simulink model "incubator_larma"  (R2023a)
settings: Solver=VariableStepAuto  StartTime=0.0  StopTime=10000  RelTol=1e-3
undefined symbols (not defined in the file or in its folder): Acv, Anet, Ar, As, Awi, bf, cp_b, cp_co, cpa, cpa_skin, cpm, cpw, eps_s, epsilon_w, Evap, hf_g, hfg, hien, hscv, IV, K_c, Kmat, kplex, m, ma, mco, ms, mw, Qmet, rho_a, rho_bl, rho_c, rho_w, Sa, sigma, th_w, thm, Wa, Wex
libraries: neural x1
settings Model: Creator=ACER  LastModifiedBy=ACER

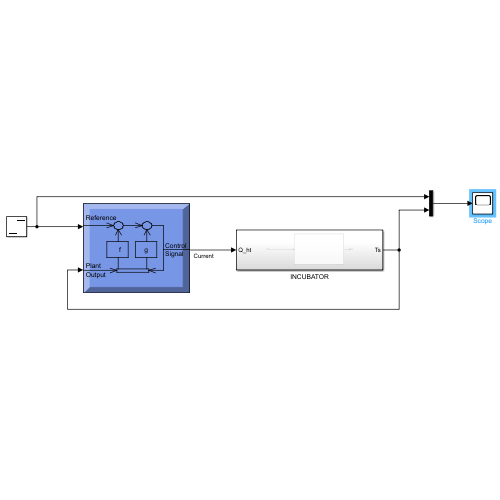
[thumbnail: Simulink's stored preview of the top-level diagram]
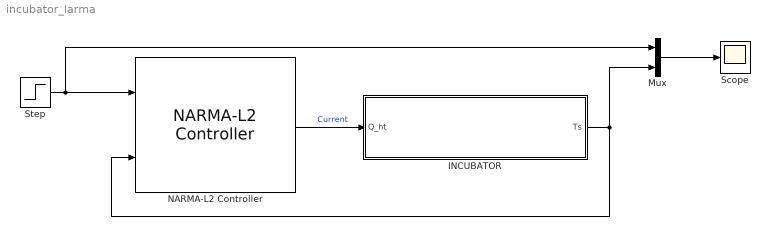
== system incubator_larma ==
  INCUBATOR : Subsystem
  Mux : Mux  Inputs=2
  NARMA-L2 Controller : neural/Control Systems/NARMA-L2 Controller  Normalize=0  IW1_1=[0.55311527878139377101 0.5598203760437183707;0.46124325685294664812 -0.0015039561193254337348;0.35378378182192637968 -0.017778723358536991511;-0.56208585013665313124 0.019429595098862040975;-0.74496852231229937491 -0.19223678100702804028;-0.18032373979217605764 -1.0804233481508331201e-05;-0.0282441180623933287 -1.9488745271411685823e-05;0.56561476199323101888 -0.048980800453075734602;-0.41624725454422795146 -2.9535601674756283214e-05;0.87246018830272520361 0.16107016027459286622;0.24117893087617620074 -0.0058257948908682806455;-0.69737494610867822864 -0.10448733539812102289;0.097948441462564567184 -0.019741652792315281251;0.57418035274274692448 -7.2088683216202652541e-05;0.5152796520885649656 -0.040344453154290062236;0.30918570905807551963 -0.021130285682796120378;-0.1040299484748695158 2.2106464471173243217e-06;-0.37176051328431147791 0.10309704107792808103;0.093748564233812642366 0.047052234342038257164;-0.54216462791611841343 -0.054531523988263504166;-0.42968180781873865914 0.055813498068482229886;0.55356647159035377026 0.04282325530096745686;0.36403213956220809022 -0.012973022507361995151;0.41088826816202883574 -0.10089012273490473304;0.46853931598860942831 -0.02420455926389125309;-0.41203096230894203922 -0.10280214872710646823;0.087678220875249249233 0.08967818975138343307;0.54183175861681087682 -0.00022750990821356916307;0.35782543615690320937 -0.041306439686633167341;0.63894568298766196701 0.14555547319291906039]  IW3_2=[-0.42869384870059590309 -0.20467390647117111868;0.54536161261206483886 0.0397307131399293606;-0.20380803372964173548 -0.093567928016329390828;-0.54440336065554817413 0.0017412995823690414175;0.41258415083026206416 -0.010924801743475522076;0.30671682947788436735 -0.0013301936152310287961;-0.30320085381841443972 0.06196663873638227904;-0.45125076837662364548 -0.0013054891628779591219;0.58589863417663268219 -0.009357661584803091126;0.22471210064158819719 0.036380518448993745539;-0.44856933606073828846 0.10557310034665394471;-0.52713778378582787365 -0.53957098764537259061;0.58612163553517704351 0.00012267588482581850409;0.20481716654358936291 0.099850170401508259177;-0.53543939332965750921 0.013380088910996708676;-0.55430247583245539911 0.00015211749869671132088;-0.060674901375614320731 0.0086928668514609716556;0.64518139636977545059 0.0055338968489383293103;-0.041112178189121904859 0.0015771853488393294297;0.069279982598140429917 0.080813967189555135917;0.0028529471897044108089 0.013322308884735010667;-0.41655325465272263763 -0.00403611729657711929;0.75859708272283676855 0.089147588049559495227;0.30545267983956803093 0.20601727557974147675;-0.55870608858082249082 0.010588837453492193699;0.074302051251215472938 0.0038643249470113908914;-0.00010236459103301481788 0.032472774763839959422;-0.23911146616137041176 0.019543603347508604895;0.084384658656527999909 -0.048307095295211939512;0.56830406068870620295 0.046981911977682609682]  IW5_3=0.093113430827311188809  LW2_1=[-1.7385414418328675179 1.185031400225210918 0.83172478025034168869 -1.4923108136193563578 0.86513570813376494684 0.55423887448822461987 -0.5403848605489650625 0.53040353884286517427 0.12742495894744695906 -2.0107365617688883752 1.7239949695213867553 1.456069982897223003 2.0136612826838233836 -1.927587542673245169 1.9384591441949254875 1.1335326599628925415 1.1219315777715177518 -1.487145524998456203 -1.9666798151412503426 1.8229411277316418527 -1.8311420627738832501 -1.3707653411339519867 1.3653022355198809468 2.1154712110253384161 1.1364878446942920931 2.1020303712400054685 -1.6675216724967341086 -0.027274724183782884934 1.3949442262661992942 -1.9913939889305762865]  LW4_3=[0.3597032512256021497 -0.63118082136266029369 0.37486171525082290223 -0.013348386024869672573 0.32965125262583028221 -0.79990641798758133074 -0.67897203390229565745 -0.18071553831118514211 0.14106801226241016955 -0.59570988892262688452 0.037331896445282973518 0.39855004856611631059 0.092510865835327929507 -0.23765480170884850653 -0.055617033718718608681 0.36860629457851767921 0.24445192286607583809 -0.37506410562211284221 0.65925844056717919361 -0.45477875753864865915 -0.30552264029698922299 -1.1194017489131884435 -0.11139933444262158091 -0.057504459052148286513 -0.25054450314805248867 -1.2495401767009046701 -0.37443973064932029038 1.4029097881644230217 0.57980235994644591102 -0.07556488017899547216]  LW5_4=-0.0053469523428589880304  LW6_5=0.97064188618752011983  LW6_2=-7.744036449301247238  B1=[-50.772852052828987723;-157.51505260377004447;-124.72206827114483474;183.33515481133116509;40.772018349078749111;57.712710053475049676;21.189182089565107958;-184.18249959630355761;135.3940445785350164;-179.3078176323155617;-85.609369809779011007;154.86499019897746621;-40.425578248012868698;-171.27574200038807817;-168.27088502237748457;-104.25105583651611596;31.911665330855385037;117.260366952972376;-18.822237201337674861;142.90914902327949676;147.83695329597799173;-160.21319473749804274;-119.03241657488929661;-165.93905598251785705;-153.45448558345208312;109.23624919968654012;-12.30327231070555527;-169.01682088309237884;-119.76762132454021526;-168.55344162205301473]  B2=-0.62656785222931232759  B3=[103.90461465914759742;-155.45897959741225236;84.188394382472665711;185.07020534665056744;-133.66035289777886419;-105.11357784470929744;113.73797811918029765;158.34818497603885135;-189.66502279116127738;-50.286835771562486741;139.27722947717367674;187.17216341294783888;-187.36774339224635355;1.9653382160202776952;171.75440875792199336;180.78060676016164621;125.84219732876395881;-182.92887583701124754;19.908028989953262311;-51.212840783719776994;7.0679985755563574656;119.33282365270373759;-159.09070986719083862;69.581948327349252281;180.45817795033127595;-51.219677154901503968;20.243727181317769492;70.90923953733859264;-56.268364735671617893;-166.94159047240137284]  B4=0.090528760253516735168  Limit_output=0  min_output=0  max_output=0  Use_Previous_Weights=1  Ts=10  S1=30  Ni=2  Nj=1  sim_file=0  trainfun=trainlm  Use_validation=0  Use_Testing=0  max_i=15000  min_i=0  max_i_int=0  min_i_int=0  sam_training=0  epochs=400  minp=30.12245687143838424  maxp=6238.3357303545271861  mint=300  maxt=6238.3357303545271861
  Scope : Scope
  Step : Step  Time=0  After=310  SampleTime=0
  wires:
  Step/1 -> NARMA-L2 Controller/1, Mux/1
  INCUBATOR/1(Ts) -> NARMA-L2 Controller/2, Mux/2
  Mux/1 -> Scope/1
  NARMA-L2 Controller/1 -> INCUBATOR/1(Q_ht)  "Current"

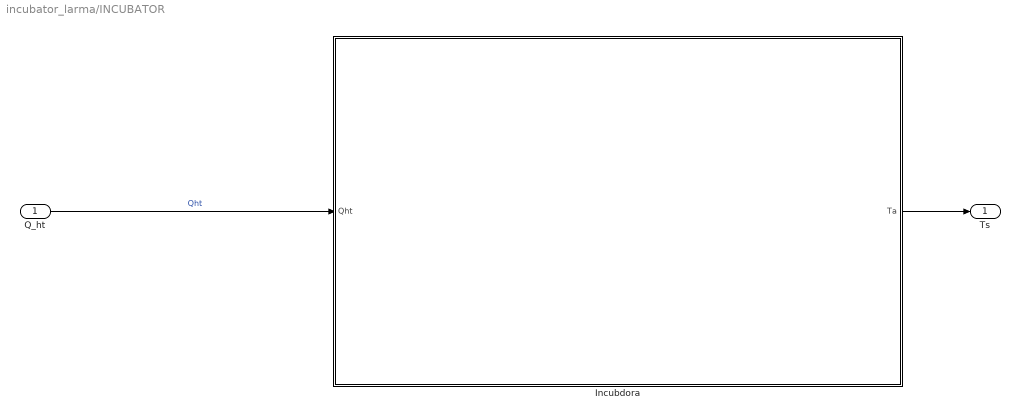
== system incubator_larma/INCUBATOR ==
  Q_ht : Inport
  Incubdora : Subsystem
  Ts : Outport
  wires:
  Q_ht/1 -> Incubdora/1(Qht)  "Qht"
  Incubdora/1(Ta) -> Ts/1

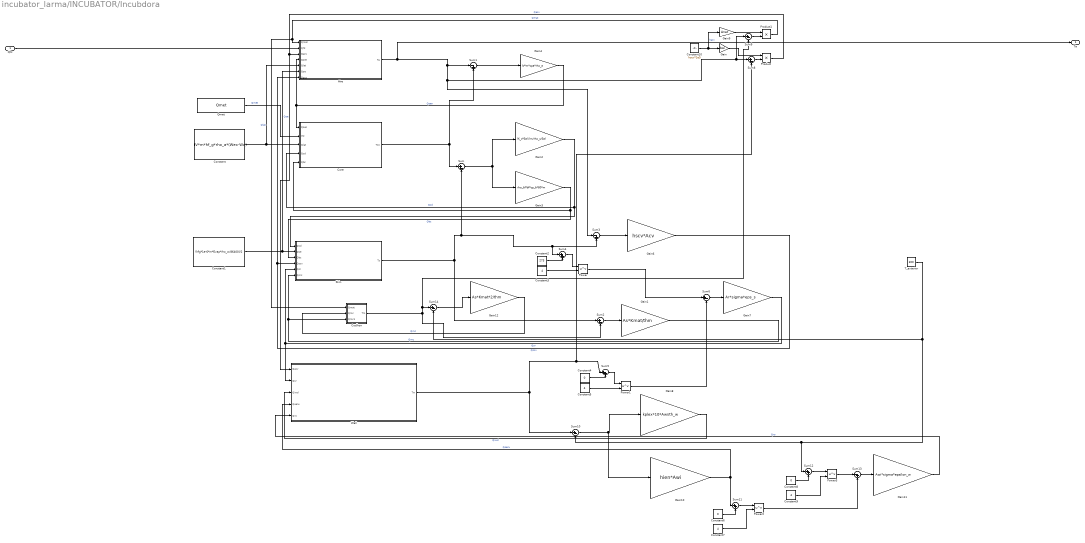
== system incubator_larma/INCUBATOR/Incubdora ==
  Qht : Inport
  Aire : Subsystem
  Coclhon : Subsystem
  Constant : Constant  Value=IV*m*hf_g*rho_a*(Wex-Wa)
  Constant1 : Constant  Value=(hfg*1e-6*m*Evap*rho_w/86400)/2
  Constant10 : Constant  Value=hscv*1e5
  Constant2 : Constant  Value=273
  Constant{3,5,7,9} (4 alike) : Constant  Value=4
  Constant4 : Constant  Value=0
  Constant6 : Constant  Value=0
  Constant8 : Constant  Value=0
  Core : Subsystem
  Gain : Gain  Gain=Awi
  Gain1 : Gain  Gain=As*Kmat/thm
  Gain10 : Gain  Gain=hien*Awi
  Gain11 : Gain  Gain=Awi*sigma*epsilon_w
  Gain12 : Gain  Gain=As*Kmat*2/thm
  Gain2 : Gain  Gain=(K_c*Sa)/(m/rho_c/Sa)
  Gain3 : Gain  Gain=rho_bl*bf*cp_b*80*m
  Gain4 : Gain  Gain=IV*m*cpa*rho_a
  Gain6 : Gain  Gain=hscv*Acv
  Gain7 : Gain  Gain=Ar*sigma*eps_s
  Gain8 : Gain  Gain=kplex*10*Awi/th_w
  Gain9 : Gain  Gain=Anet
  Power{,1..3} (4 alike) : Math  Operator=pow
  Product : Product
  Product1 : Product
  Qmet : Constant  Value=Qmet
  Skin : Subsystem
  Sum{,2,6,8..10,14} (7 alike) : Sum  Inputs=|+-
  Sum1 : Sum  Inputs=|-+
  Sum{4..5,11..12} (4 alike) : Sum  Inputs=|++
  Sum13 : Sum  Inputs=|-+
  Sum3 : Sum  Inputs=|-+
  T_exterior : Constant  Value=300
  Wall : Subsystem
  Ta : Outport
  wires:
  Product1/1 -> Coclhon/1(Qmat), Aire/1(Qmat)  "Qmat"
  Gain8/1 -> Wall/3(Qiwd)  "Qiwd"
  Product/1 -> Wall/1(Qacv), Aire/3(Qacv)  "Qacv"
  Power/1 -> Sum6/1
  Gain2/1 -> Skin/1(Qcd), Core/4(Qcd)  "Qcd"
  Sum1/1 -> Gain4/1
  Constant3/1 -> Power/2
  Aire/1(Ta) -> Ta/1, Sum9/1, Sum8/1, Sum3/1, Sum1/1
  Qmet/1 -> Core/2(In2)  "Qmet"
  Power1/1 -> Sum6/2
  Sum4/1 -> Power/1
  Sum3/1 -> Gain6/1
  Sum14/1 -> Gain12/1
  Coclhon/1(Tm) -> Sum2/2, Sum14/1, Sum9/2
  Sum5/1 -> Power1/1
  Constant2/1 -> Sum4/2
  Gain7/1 -> Wall/2(Qsr), Skin/5(Qsr)  "Qsr"
  Gain4/1 -> Aire/4(Qsen), Core/1(Qsen)  "Qsen"
  Constant1/1 -> Aire/6(Qse), Skin/2(Qse)  "Qse"
  Sum/1 -> Gain3/1, Gain2/1
  Gain11/1 -> Wall/5(Qro)  "Qro"
  Sum13/1 -> Gain11/1
  Constant8/1 -> Sum12/2
  Gain9/1 -> Product1/1
  Gain1/1 -> Skin/6(Qmc), Coclhon/3(Qmc1)  "Qmc"
  Core/1(Tco) -> Sum1/2, Sum/1
  Constant4/1 -> Sum5/2
  Wall/1(Tw) -> Sum8/2, Sum5/1, Sum10/1
  Skin/1(Ts) -> Sum4/1, Sum3/2, Sum/2, Sum2/1
  Constant5/1 -> Power1/2
  Constant6/1 -> Sum11/2
  Sum2/1 -> Gain1/1
  Gain/1 -> Product/1
  Constant10/1 -> Gain9/1, Gain/1  "hacv"
  Gain6/1 -> Aire/7(Qscv), Skin/4(Qscv)  "Qscv"
  Gain3/1 -> Skin/3(Qbc), Core/5(Qbc)  "Qbc"
  Sum8/1 -> Product/2
  Gain10/1 -> Wall/4(Qoenv), Sum11/1  "Qoenv"
  Power2/1 -> Sum13/2
  T_exterior/1 -> Sum14/2, Sum12/1, Sum10/2
  Sum12/1 -> Power3/1
  Gain12/1 -> Coclhon/2(Qmc)  "Qmc"
  Sum10/1 -> Gain10/1, Gain8/1
  Constant7/1 -> Power2/2
  Constant9/1 -> Power3/2
  Sum6/1 -> Gain7/1
  Sum9/1 -> Product1/2
  Sum11/1 -> Power2/1
  Power3/1 -> Sum13/1
  Constant/1 -> Aire/5(Qlat), Core/3(Qlat)  "Qlat"
  Qht/1 -> Aire/2(Qht)

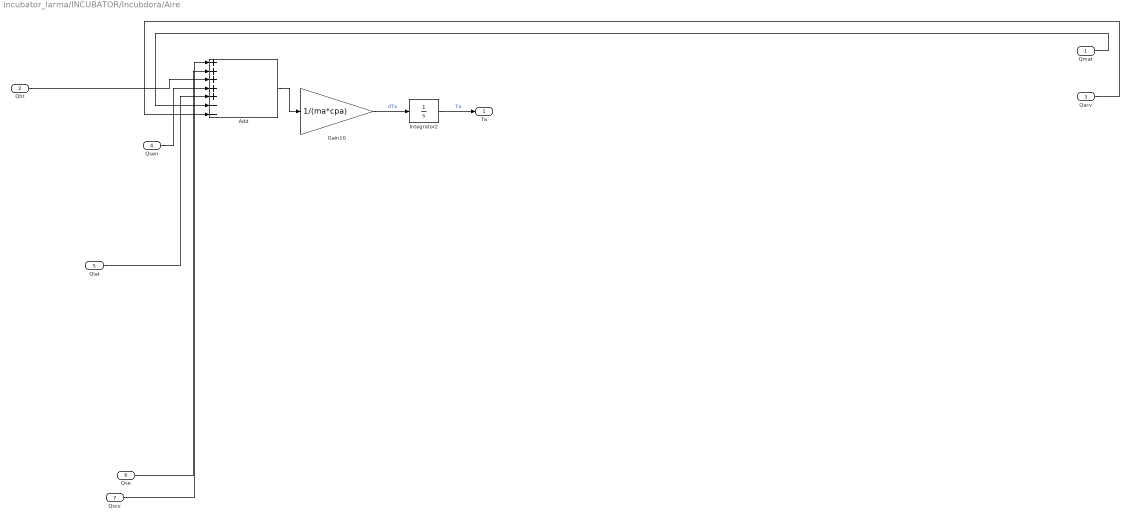
== system incubator_larma/INCUBATOR/Incubdora/Aire ==
  Qmat : Inport
  Qht : Inport  Port=2
  Qacv : Inport  Port=3
  Qsen : Inport  Port=4
  Qlat : Inport  Port=5
  Qse : Inport  Port=6
  Qscv : Inport  Port=7
  Add : Sum  Inputs=+++++--
  Gain10 : Gain  Gain=1/(ma*cpa)
  Integrator2 : Integrator  InitialCondition=300
  Ta : Outport
  wires:
  Qse/1 -> Add/2
  Qsen/1 -> Add/4
  Qlat/1 -> Add/5
  Add/1 -> Gain10/1
  Integrator2/1 -> Ta/1  "Ta"
  Gain10/1 -> Integrator2/1  "dTa"
  Qht/1 -> Add/3
  Qscv/1 -> Add/1
  Qacv/1 -> Add/7
  Qmat/1 -> Add/6

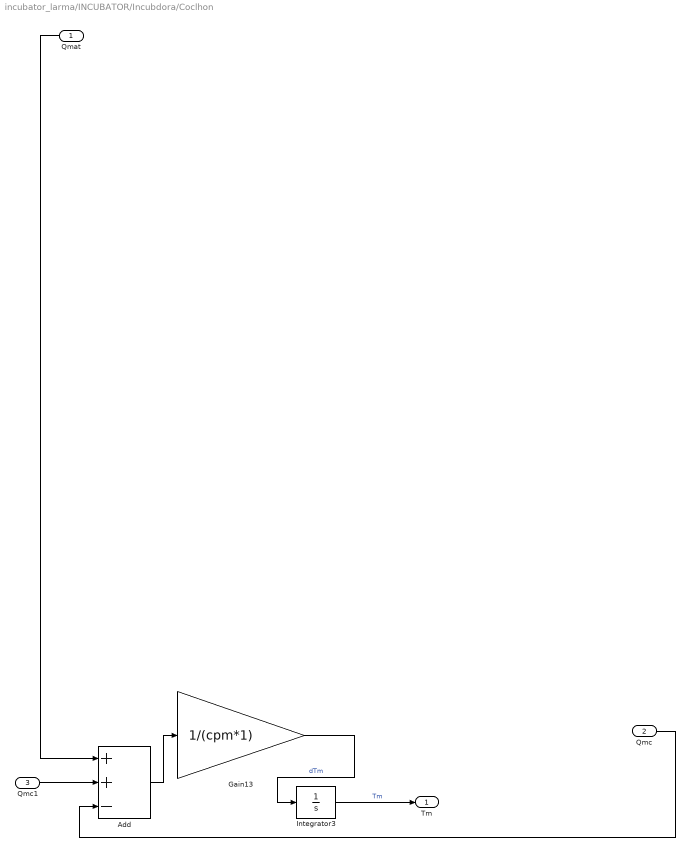
== system incubator_larma/INCUBATOR/Incubdora/Coclhon ==
  Qmat : Inport
  Qmc : Inport  Port=2
  Qmc1 : Inport  Port=3
  Add : Sum  Inputs=++-
  Gain13 : Gain  Gain=1/(cpm*1)
  Integrator3 : Integrator  InitialCondition=308
  Tm : Outport
  wires:
  Integrator3/1 -> Tm/1  "Tm"
  Add/1 -> Gain13/1
  Gain13/1 -> Integrator3/1  "dTm"
  Qmc/1 -> Add/3
  Qmat/1 -> Add/1
  Qmc1/1 -> Add/2

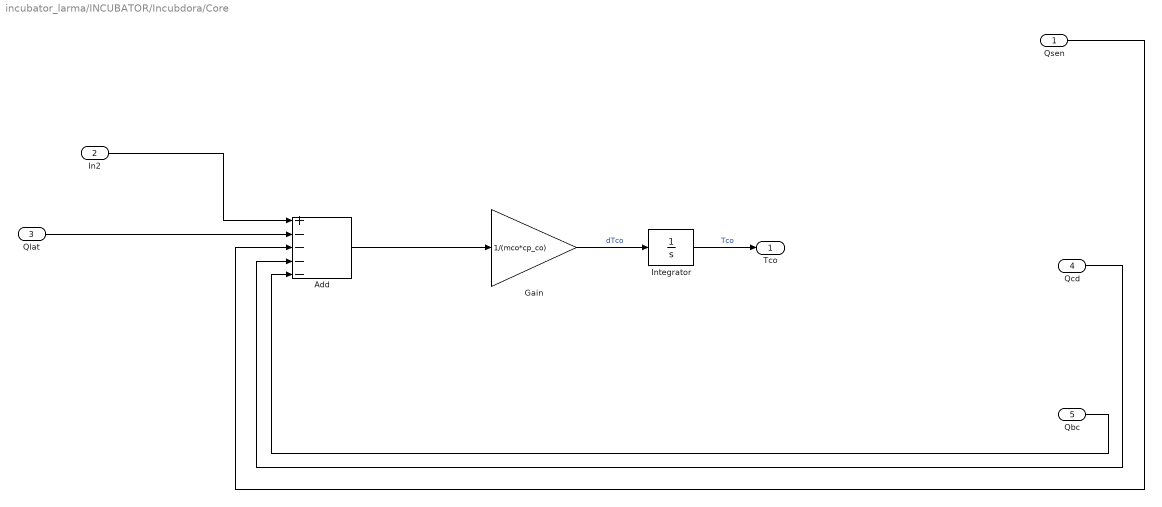
== system incubator_larma/INCUBATOR/Incubdora/Core ==
  Qsen : Inport
  In2 : Inport  Port=2
  Qlat : Inport  Port=3
  Qcd : Inport  Port=4
  Qbc : Inport  Port=5
  Add : Sum  Inputs=+----
  Gain : Gain  Gain=1/(mco*cp_co)
  Integrator : Integrator  InitialCondition=308
  Tco : Outport
  wires:
  Qlat/1 -> Add/2
  Gain/1 -> Integrator/1  "dTco"
  Qbc/1 -> Add/5
  Qcd/1 -> Add/4
  Integrator/1 -> Tco/1  "Tco"
  Add/1 -> Gain/1
  In2/1 -> Add/1
  Qsen/1 -> Add/3

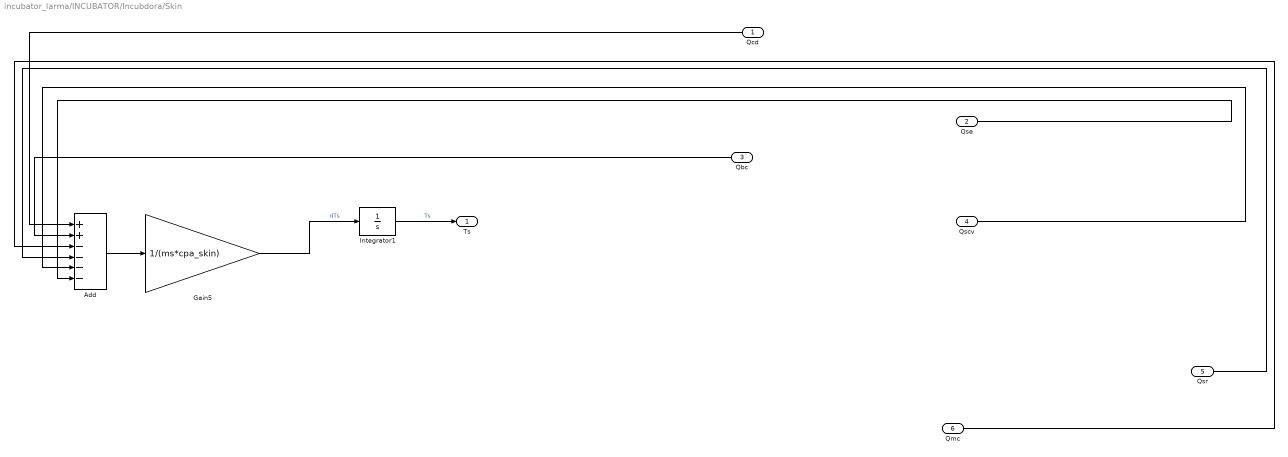
== system incubator_larma/INCUBATOR/Incubdora/Skin ==
  Qcd : Inport
  Qse : Inport  Port=2
  Qbc : Inport  Port=3
  Qscv : Inport  Port=4
  Qsr : Inport  Port=5
  Qmc : Inport  Port=6
  Add : Sum  Inputs=++----
  Gain5 : Gain  Gain=1/(ms*cpa_skin)
  Integrator1 : Integrator  InitialCondition=308
  Ts : Outport
  wires:
  Qbc/1 -> Add/2
  Qscv/1 -> Add/5
  Add/1 -> Gain5/1
  Gain5/1 -> Integrator1/1  "dTs"
  Qse/1 -> Add/6
  Qmc/1 -> Add/3
  Qsr/1 -> Add/4
  Integrator1/1 -> Ts/1  "Ts"
  Qcd/1 -> Add/1

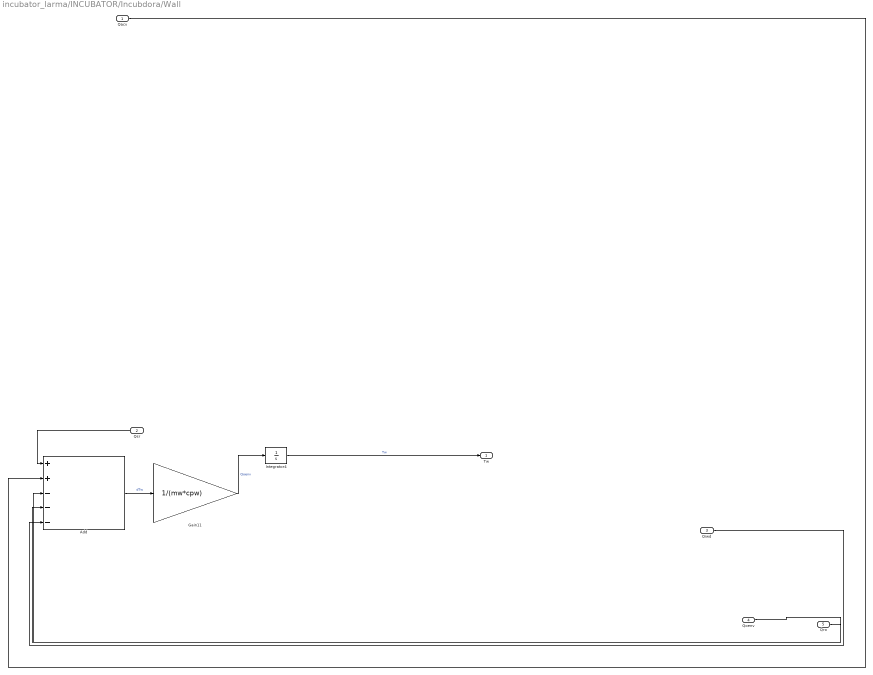
== system incubator_larma/INCUBATOR/Incubdora/Wall ==
  Qacv : Inport
  Qsr : Inport  Port=2
  Qiwd : Inport  Port=3
  Qoenv : Inport  Port=4
  Qro : Inport  Port=5
  Add : Sum  Inputs=++---
  Gain11 : Gain  Gain=1/(mw*cpw)
  Integrator4 : Integrator  InitialCondition=308
  Tw : Outport
  wires:
  Add/1 -> Gain11/1  "dTw"
  Qsr/1 -> Add/1
  Qacv/1 -> Add/2
  Gain11/1 -> Integrator4/1  "Qoenv"
  Qoenv/1 -> Add/4
  Qiwd/1 -> Add/5
  Qro/1 -> Add/3
  Integrator4/1 -> Tw/1  "Tw"
